simulink model "BusDirectPorts"  (Simulink 7.4)
settings: Solver=ode45  StartTime=0.0  StopTime=10.0  RelTol=1e-3
PostLoadFcn:
  | load Bus.mat
settings Model: Creator=dread  LastModifiedBy=dread

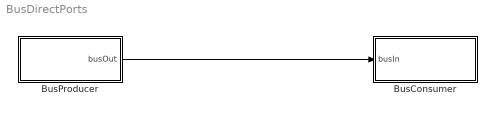
== system BusDirectPorts ==
  BusConsumer : Subsystem
  BusProducer : Subsystem
  wires:
  BusProducer/1(busOut) -> BusConsumer/1(busIn)

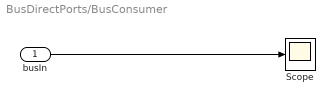
== system BusDirectPorts/BusConsumer ==
  busIn : Inport  UseBusObject=on  OutDataType=fixdt(1, 16)  OutScaling=2^0
      settings: BusObject=Bus
  Scope : Scope
  wires:
  busIn/1 -> Scope/1

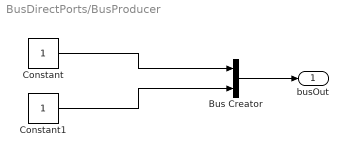
== system BusDirectPorts/BusProducer ==
  Bus Creator : BusCreator  Inputs=2  UseBusObject=on
      settings: BusObject=Bus
  Constant : Constant  OutDataType=fixdt(1, 16)  OutScaling=2^0
  Constant1 : Constant  OutDataType=fixdt(1, 16)  OutScaling=2^0
  busOut : Outport  UseBusObject=on  OutDataType=fixdt(1, 16)  OutScaling=2^0
      settings: BusObject=Bus
  wires:
  Bus Creator/1 -> busOut/1
  Constant/1 -> Bus Creator/1
  Constant1/1 -> Bus Creator/2
